simulink model "mintamodell"  (Simulink 6.1)
settings: Solver=ode14x  StartTime=0.0  StopTime=100  FixedStep=0.2  RelTol=1e-3
libraries: simulink x4
settings Model: Creator=MUNKA  LastModifiedBy=Labor
settings DebuggingCC: SolverPrmCheckMsg=warning

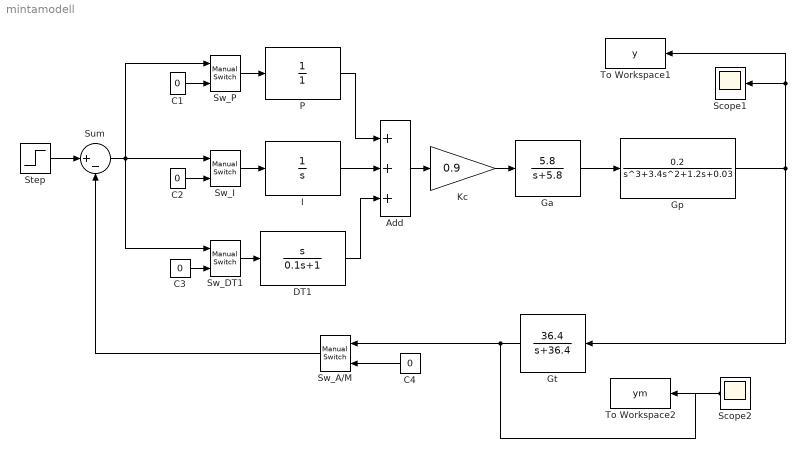
== system mintamodell ==
  " Sw_A/M" : simulink/Signal Routing/Manual Switch  Orientation=left  sw=1  action=0
  " Sw_DT1" : simulink/Signal Routing/Manual Switch  sw=0  action=0
  Add : Sum  Inputs=+++  OutScaling=2^-10
  C1 : Constant  Value=0
  C2 : Constant  Value=0
  C3 : Constant  Value=0
  C4 : Constant  Orientation=left  Value=0
  DT1 : TransferFcn  Numerator=[1 0]  Denominator=[0.1 1]
  "Ga " : TransferFcn  Numerator=[5.8]  Denominator=[1 5.8]
  Gp : TransferFcn  Numerator=[0.2]  Denominator=[1 3.4 1.2 0.03]
  Gt : TransferFcn  Orientation=left  Numerator=[36.4]  Denominator=[1 36.4]
  I : TransferFcn  Denominator=[1 0 ]
  Kc : Gain  Gain=0.9
  P : TransferFcn  Denominator=[1 ]
  Scope1 : Scope
  Scope2 : Scope
  Step : Step  Time=0  SampleTime=0
  Sum : Sum  Inputs=|+-
  Sw_I : simulink/Signal Routing/Manual Switch  sw=0  action=0
  Sw_P : simulink/Signal Routing/Manual Switch  sw=1  action=0
  To Workspace1 : ToWorkspace  VariableName=y  SampleTime=-1  SaveFormat=Array
  To Workspace2 : ToWorkspace  VariableName=ym  SampleTime=-1  SaveFormat=Array
  wires:
  Sw_I/1 -> I/1
  " Sw_DT1"/1 -> DT1/1
  I/1 -> Add/2
  DT1/1 -> Add/3
  Add/1 -> Kc/1
  Gp/1 -> Gt/1, Scope1/1, To Workspace1/1
  Sum/1 -> Sw_I/1, " Sw_DT1"/1, Sw_P/1
  Step/1 -> Sum/1
  C2/1 -> Sw_I/2
  C3/1 -> " Sw_DT1"/2
  C4/1 -> " Sw_A/M"/2
  "Ga "/1 -> Gp/1
  Kc/1 -> "Ga "/1
  " Sw_A/M"/1 -> Sum/2
  P/1 -> Add/1
  Gt/1 -> " Sw_A/M"/1, Scope2/1, To Workspace2/1
  C1/1 -> Sw_P/2
  Sw_P/1 -> P/1
